simulink model "decoder"  (R2012b)
settings: Solver=FixedStepDiscrete  StartTime=0.0  StopTime=10.0  FixedStep=0.001  RelTol=1e-3
undefined symbols (not defined in the file): A, biasCorrectionEnable, biasCorrectionInitial, biasCorrectionPower, biasCorrectionResetToInitial, biasCorrectionStateInds, biasCorrectionTau, biasCorrectionType, biasCorrectionVelocityThreshold, C, Cfeedback, continuousEnable, DecoderConstants, decoderType, discreteEnable, discreteFilterName, discreteInvSoftNormVals, discretePcaMeans, discreteProjector, dtMS, filterName, gainK, hLFPDivisor, hLFPTransform, hmmEmisCovarDet, hmmEmisCovarInv, hmmEmisMean, hmmNumStates, hmmSpeedScalingBins, hmmSpeedScalingEnable, hmmSpeedScalingPs, hmmStateModel, hmmTrans, invSoftNormVals, K, meansTrackingEnable, meansTrackingInitial, meansTrackingPeriodMS, meansTrackingResetToCurrent, meansTrackingResetToInitial, meansTrackingUseFastAdapt, offsetXk, pcaMeans, projector, scaleXk, smoothingKernel, spikeTransform, thresholds, useAcaus, xkConstants
settings Model: xpc_rtwmakecfg_data=_xpcetherlib__xpcether8255xlib__xpcetherGbElib__xpcnblib_  Creator=gilja  LastModifiedBy=NPTL
settings SolverCC: EnableConcurrentExecution=on  ConcurrentTasks=on
settings DataIOCC: LimitDataPoints=off  SaveOutput=off  SaveTime=off
settings OptimizationCC: InlineParams=on  InlineInvariantSignals=on  EnhancedBackFolding=on  EfficientFloat2IntCast=on  SimCompilerOptimization=On
settings DebuggingCC: IntegerOverflowMsg=none
settings HardwareCC: ProdIntDivRoundTo=Zero  ProdEndianess=LittleEndian  ProdHWDeviceType=Generic->32-bit x86 compatible
settings ModelReferenceCC: ModelReferenceNumInstancesAllowed=Single  ModelReferenceMinAlgLoopOccurrences=on
settings RTWCC: SystemTargetFile=xpctarget.tlc  TemplateMakefile=xpc_default_tmf  Description=xPC Target  ProcessScript=xpctarget_make_rtw_hook  RTWCompilerOptimization=On  RTWCustomCompilerOptimizations=-O fold_scalar_mxarrays:on -O fold_non_scalar_mxarrays:on -O array_indexing:on -O optimize_integer_for_loops:on -O optimize_conditionals:on
settings CodeAppCC: MaxIdLength=62
settings xpcTargetCC: TargetFcnLib=ansi_tfl_table_tmw.mat  CodeReplacementLibrary=XPC_BLAS  ParMdlRefBuildCompliant=on  ConcurrentExecutionCompliant=on  CombineSignalStateStructs=off  GRTInterface=on  ExtMode=off  xPCTaskExecutionProfile=on  xPCRL32EventNumber=5000  xPCisDownloadable=off  xPCLoadParamSetFile=off  xPCConcurrentTasks=off  xPCEnableSFAnimation=off

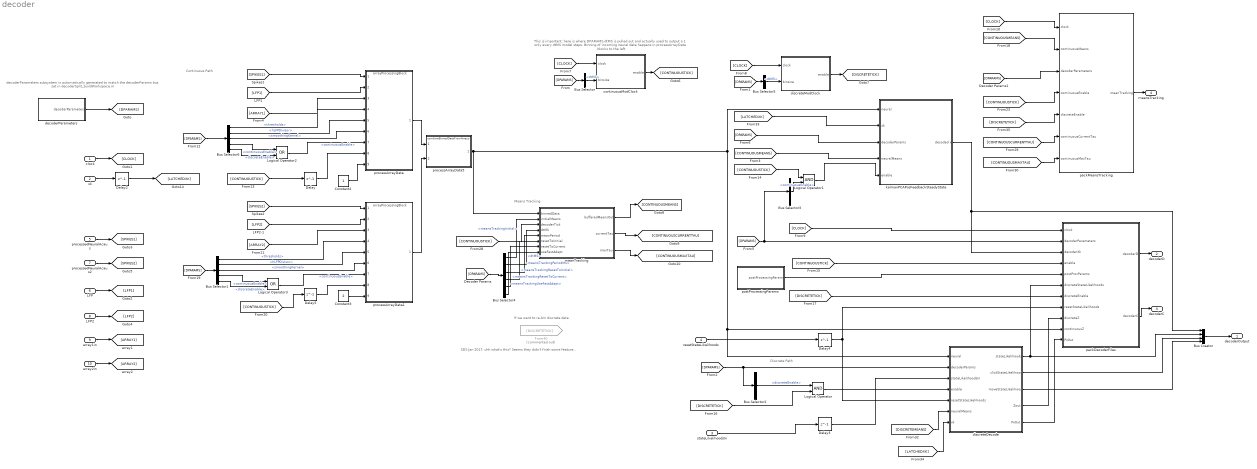
== system decoder ==
  note: SDS Jan 2017: uhh what's this? Seems they didn't fnish some feature...
  note: This is important: here is where DPARAMS.dtMS is pulled out and actually used to
      | output a 1 only every dtMS model steps. Binning of incoming neural data happens in
      | processArrayData blocks to the left
  note: Means Tracking
  note: decoderParameters subsystem is
      |  automatically generated to match the decoderParams
      | bus set in decoderSplit_buildWorkspace.m
  note: Discrete Path
  note: Continuous Path
  note: If we want to re-bin discrete data
  clock : Inport  OutDataTypeStr=uint32
  xk : Inport  Port=2  OutDataTypeStr=double  PortDimensions=[double(xkConstants.NUM_STATE_DIMENSIONS),1]
  stateLikelihoodsIn : Inport  Port=3  OutDataTypeStr=double  PortDimensions=[double(DecoderConstants.MAX_DISCRETE_STATES) 1]
  resetStateLikelihoods : Inport  Port=4  OutDataTypeStr=double  PortDimensions=1
  processedNeuralAcaus : Inport  Port=5  OutDataTypeStr=Bus: processedNeural  BusOutputAsStruct=on
  LFP : Inport  Port=6  OutDataTypeStr=single  PortDimensions=[1 96]
  processedNeuralAcaus2 : Inport  Port=7  OutDataTypeStr=Bus: processedNeural  BusOutputAsStruct=on
  LFP2 : Inport  Port=8  OutDataTypeStr=single  PortDimensions=[1 96]
  array1in : Inport  Port=9  OutDataTypeStr=uint8  BusOutputAsStruct=on
  array2in : Inport  Port=10  OutDataTypeStr=uint8  BusOutputAsStruct=on
  Bus Creator : BusCreator  OutDataTypeStr=Bus: decoderOutput  NonVirtualBus=on
  Bus Selector : BusSelector  OutputSignals=dtMS
  Bus Selector1 : BusSelector  OutputSignals=thresholds,hLFPDivisor,smoothingKernel,continuousEnable,discreteEnable
  Bus Selector2 : BusSelector  OutputSignals=discreteEnable
  Bus Selector3 : BusSelector  OutputSignals=continuousEnable
  Bus Selector4 : BusSelector  OutputSignals=meansTrackingInitial,dtMS,meansTrackingPeriodMS,meansTrackingResetToInitial,meansTrackingResetToCurrent,meansTrackingUseFastAdapt
  Bus Selector5 : BusSelector  OutputSignals=dtMS
  Bus Selector6 : BusSelector  OutputSignals=thresholds,hLFPDivisor,smoothingKernel,continuousEnable,discreteEnable
  Constant2 : Constant  VectorParams1D=off  SampleTime=-1
  Constant3 : Constant  Value=2  VectorParams1D=off  SampleTime=-1
  Delay{,2..5} (5 alike) : Delay  DelayLength=1
  From40 : From  Commented=on  GotoTag=DISCRETETICK
  Logical Operator : Logic  AllPortsSameDT=off  OutDataTypeStr=boolean
  Logical Operator1 : Logic  AllPortsSameDT=off  OutDataTypeStr=boolean
  Logical Operator2 : Logic  Operator=OR  AllPortsSameDT=off  OutDataTypeStr=boolean
  Logical Operator3 : Logic  Operator=OR  AllPortsSameDT=off  OutDataTypeStr=boolean
  continuousModClock : MATLAB Function  TreatAsAtomicUnit=on
  decoderParameters : Subsystem
  discreteDecode : Subsystem
  discreteModClock : MATLAB Function  TreatAsAtomicUnit=on
  kalmanPCAPosFeedbackSteadyState : Subsystem
  meanTracking : MATLAB Function  TreatAsAtomicUnit=on
  packDecoderFiles : MATLAB Function  TreatAsAtomicUnit=on
  packMeansTracking : MATLAB Function  TreatAsAtomicUnit=on
  postProcessingParams : Subsystem
  processArrayData : ModelReference  ModelNameDialog=arrayProcessingBlock  SimulationMode=Normal  ModelReferenceVersion=1.56  CopyOfModelName=arrayProcessingBlock  DefaultDataLogging=on
  processArrayData1 : ModelReference  ModelNameDialog=arrayProcessingBlock  SimulationMode=Normal  ModelReferenceVersion=1.56  CopyOfModelName=arrayProcessingBlock  DefaultDataLogging=on
  processArrayData5 : ModelReference  ModelNameDialog=combineBinnedDataFromArrays  SimulationMode=Normal  ModelReferenceVersion=1.49  CopyOfModelName=combineBinnedDataFromArrays  DefaultDataLogging=on
  decoderOutput : Outport  OutDataTypeStr=Bus: decoderOutput  BusOutputAsStruct=on
  decoderD : Outport  Port=2  OutDataTypeStr=Bus: fileLoggerFormatAndData  BusOutputAsStruct=on
  decoderC : Outport  Port=3  OutDataTypeStr=Bus: fileLoggerFormatAndData  BusOutputAsStruct=on
  meansTracking : Outport  Port=4  OutDataTypeStr=Bus: fileLoggerFormatAndData  BusOutputAsStruct=on
  wires:
  Bus Selector/1 -> continuousModClock/2(binsize)  "<dtMS>"
  [LATCHEDXK] -> kalmanPCAPosFeedbackSteadyState/2(xk)
  decoderParameters/1(decoderParameters) -> [DPARAMS]
  discreteDecode/1(stateLikelihoods) -> Bus Creator/2, packDecoderFiles/6(discreteStateLikelihoods)
  Bus Creator/1 -> decoderOutput/1
  stateLikelihoodsIn/1 -> Delay3/1
  Delay3/1 -> discreteDecode/3(stateLikelihoodsIn)
  discreteDecode/2(clickStateLikelihood) -> Bus Creator/3
  discreteDecode/3(moveStateLikelihood) -> Bus Creator/4
  Delay4/1 -> discreteDecode/5(resetStateLikelihoods), packDecoderFiles/8(resetStateLikelihoods)
  resetStateLikelihoods/1 -> Delay4/1
  [DPARAMS] -> Bus Selector/1
  [DPARAMS] -> Bus Selector2/1, discreteDecode/2(decoderParams)
  [DPARAMS] -> kalmanPCAPosFeedbackSteadyState/3(decoderParams)
  clock/1 -> [CLOCK]
  [CLOCK] -> continuousModClock/1(clock)
  [CLOCK] -> packDecoderFiles/1(clock)
  LFP/1 -> [LFP1]
  processedNeuralAcaus/1 -> [SPIKES1]
  discreteDecode/4(Zout) -> packDecoderFiles/9(discreteZ)
  LFP2/1 -> [LFP2]
  processedNeuralAcaus2/1 -> [SPIKES2]
  array1in/1 -> [ARRAY1]
  array2in/1 -> [ARRAY2]
  [DPARAMS] -> Bus Selector6/1
  [SPIKES1] -> processArrayData/1
  [LFP1] -> processArrayData/2
  Bus Selector6/2 -> processArrayData/5  "<hLFPDivisor>"
  Bus Selector6/3 -> processArrayData/6  "<smoothingKernel>"
  Delay/1 -> processArrayData/8
  [ARRAY1] -> processArrayData/3
  continuousModClock/1(enable) -> [CONTINUOUSTICK]
  [CONTINUOUSTICK] -> Delay/1
  [CONTINUOUSTICK] -> packDecoderFiles/4(enable)
  Logical Operator/1 -> discreteDecode/4(enable)
  [DISCRETETICK] -> packDecoderFiles/7(discreteEnable)
  [DPARAMS] -> Bus Selector1/1
  [SPIKES2] -> processArrayData1/1
  [LFP2] -> processArrayData1/2
  Bus Selector1/2 -> processArrayData1/5  "<hLFPDivisor>"
  Bus Selector1/3 -> processArrayData1/6  "<smoothingKernel>"
  Delay5/1 -> processArrayData1/8
  [ARRAY2] -> processArrayData1/3
  [CONTINUOUSTICK] -> Delay5/1
  processArrayData/1 -> processArrayData5/1
  processArrayData1/1 -> processArrayData5/2
  Constant2/1 -> processArrayData/9
  Bus Selector6/1 -> processArrayData/4  "<thresholds>"
  Bus Selector1/1 -> processArrayData1/4  "<thresholds>"
  Constant3/1 -> processArrayData1/9
  [CLOCK] -> discreteModClock/1(clock)
  discreteModClock/1(enable) -> [DISCRETETICK]
  Logical Operator3/1 -> processArrayData1/7  "<continuousEnable>"
  Logical Operator2/1 -> processArrayData/7  "<continuousEnable>"
  [DISCRETETICK] -> Logical Operator/2
  Bus Selector2/1 -> Logical Operator/1  "<discreteEnable>"
  Bus Selector3/1 -> Logical Operator1/2  "<continuousEnable>"
  Logical Operator1/1 -> kalmanPCAPosFeedbackSteadyState/5(enable)
  [CONTINUOUSTICK] -> Logical Operator1/1
  [DPARAMS] -> Bus Selector3/1, packDecoderFiles/2(decoderParameters)
  [DPARAMS] -> Bus Selector4/1
  Bus Selector4/2 -> meanTracking/4(dtMS)  "<dtMS>"
  Bus Selector4/1 -> meanTracking/2(initialMeans)  "<meansTrackingInitial>"
  meanTracking/1(bufferedMeansOut) -> [CONTINUOUSMEANS]
  [CONTINUOUSMEANS] -> kalmanPCAPosFeedbackSteadyState/4(neuralMeans)
  [CLOCK] -> packMeansTracking/1(clock)
  [DPARAMS] -> packMeansTracking/3(decoderParameters)
  [CONTINUOUSMEANS] -> packMeansTracking/2(continuousMeans)
  [CONTINUOUSTICK] -> packMeansTracking/4(continuousEnable)
  [CONTINUOUSTICK] -> meanTracking/3(decoderTick)
  Bus Selector4/3 -> meanTracking/5(meanPeriod)  "<meansTrackingPeriodMS>"
  Bus Selector4/4 -> meanTracking/6(resetToInitial)  "<meansTrackingResetToInitial>"
  Bus Selector4/5 -> meanTracking/7(resetToCurrent)  "<meansTrackingResetToCurrent>"
  Bus Selector4/6 -> meanTracking/8(useFastAdapt)  "<meansTrackingUseFastAdapt>"
  meanTracking/2(currentTau) -> [CONTINUOUSCURRENTTAU]
  meanTracking/3(maxTau) -> [CONTINUOUSMAXTAU]
  [CONTINUOUSMAXTAU] -> packMeansTracking/7(continuousMaxTau)
  [CONTINUOUSCURRENTTAU] -> packMeansTracking/6(continuousCurrentTau)
  processArrayData5/1 -> meanTracking/1(binnedData), discreteDecode/1(neural), packDecoderFiles/10(continuousZ), kalmanPCAPosFeedbackSteadyState/1(neural)
  [DISCRETEMEANS] -> discreteDecode/6(neuralMeans)
  [LATCHEDXK] -> discreteDecode/7(xk)
  Delay2/1 -> [LATCHEDXK]
  xk/1 -> Delay2/1
  [DISCRETETICK] -> packMeansTracking/5(discreteEnable)
  kalmanPCAPosFeedbackSteadyState/1(decoded x) -> packDecoderFiles/3(decoderXk), Bus Creator/1
  Bus Selector6/4 -> Logical Operator2/1  "<continuousEnable>"
  Bus Selector6/5 -> Logical Operator2/2  "<discreteEnable>"
  Bus Selector1/4 -> Logical Operator3/1  "<continuousEnable>"
  Bus Selector1/5 -> Logical Operator3/2  "<discreteEnable>"
  packMeansTracking/1(meanTracking) -> meansTracking/1
  packDecoderFiles/2(decoderC) -> decoderC/1
  packDecoderFiles/1(decoderD) -> decoderD/1
  Bus Selector5/1 -> discreteModClock/2(binsize)  "<dtMS>"
  [DPARAMS] -> Bus Selector5/1
  discreteDecode/5(PxOut) -> packDecoderFiles/11(PxOut)
  postProcessingParams/1(postProcessingParams) -> packDecoderFiles/5(postProcParams)

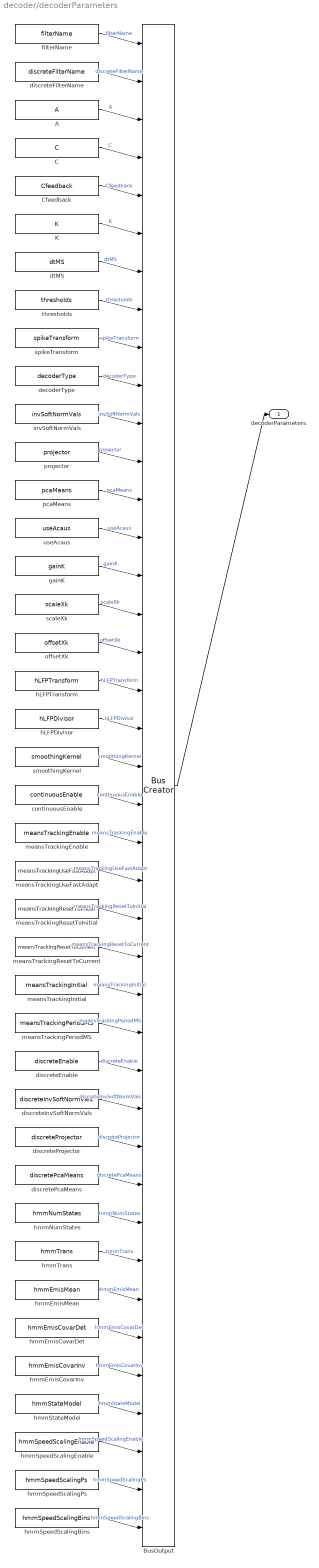
== system decoder/decoderParameters ==
  A : Constant  Value=A
  BusOutput : BusCreator  Inputs=filterName,discreteFilterName,A,C,Cfeedback,K,dtMS,thresholds,spikeTransform,decoderType,invSoftNormVals,projector,pcaMeans,useAcaus,gainK,scaleXk,offsetXk,hLFPTransform,hLFPDivisor,smoothingKernel,continuousEnable,meansTrackingEnable,meansTrackingUseFastAdapt,meansTrackingResetToInitial,meansTrackingResetToCurrent,meansTrackingInitial,meansTrackingPeriodMS,discreteEnable,discreteInvSoftNormVals,discreteProjector,discretePcaMeans,hmmNumStates,hmmTrans,hmmEmisMean,hmmEmisCovarDet,hmmEmisCovarInv,hmmStateModel,hmmSpeedScalingEnable,hmmSpeedScalingPs,hmmSpeedScalingBins  OutDataTypeStr=Bus: decoderParams
  C : Constant  Value=C
  Cfeedback : Constant  Value=Cfeedback
  K : Constant  Value=K
  continuousEnable : Constant  Value=continuousEnable
  decoderType : Constant  Value=decoderType
  discreteEnable : Constant  Value=discreteEnable
  discreteFilterName : Constant  Value=discreteFilterName
  discreteInvSoftNormVals : Constant  Value=discreteInvSoftNormVals
  discretePcaMeans : Constant  Value=discretePcaMeans
  discreteProjector : Constant  Value=discreteProjector
  dtMS : Constant  Value=dtMS
  filterName : Constant  Value=filterName
  gainK : Constant  Value=gainK
  hLFPDivisor : Constant  Value=hLFPDivisor
  hLFPTransform : Constant  Value=hLFPTransform
  hmmEmisCovarDet : Constant  Value=hmmEmisCovarDet
  hmmEmisCovarInv : Constant  Value=hmmEmisCovarInv
  hmmEmisMean : Constant  Value=hmmEmisMean
  hmmNumStates : Constant  Value=hmmNumStates
  hmmSpeedScalingBins : Constant  Value=hmmSpeedScalingBins
  hmmSpeedScalingEnable : Constant  Value=hmmSpeedScalingEnable
  hmmSpeedScalingPs : Constant  Value=hmmSpeedScalingPs
  hmmStateModel : Constant  Value=hmmStateModel
  hmmTrans : Constant  Value=hmmTrans
  invSoftNormVals : Constant  Value=invSoftNormVals
  meansTrackingEnable : Constant  Value=meansTrackingEnable
  meansTrackingInitial : Constant  Value=meansTrackingInitial
  meansTrackingPeriodMS : Constant  Value=meansTrackingPeriodMS
  meansTrackingResetToCurrent : Constant  Value=meansTrackingResetToCurrent
  meansTrackingResetToInitial : Constant  Value=meansTrackingResetToInitial
  meansTrackingUseFastAdapt : Constant  Value=meansTrackingUseFastAdapt
  offsetXk : Constant  Value=offsetXk
  pcaMeans : Constant  Value=pcaMeans
  projector : Constant  Value=projector
  scaleXk : Constant  Value=scaleXk
  smoothingKernel : Constant  Value=smoothingKernel
  spikeTransform : Constant  Value=spikeTransform
  thresholds : Constant  Value=thresholds
  useAcaus : Constant  Value=useAcaus
  decoderParameters : Outport
  wires:
  filterName/1 -> BusOutput/1  "filterName"
  discreteFilterName/1 -> BusOutput/2  "discreteFilterName"
  A/1 -> BusOutput/3  "A"
  C/1 -> BusOutput/4  "C"
  Cfeedback/1 -> BusOutput/5  "Cfeedback"
  K/1 -> BusOutput/6  "K"
  dtMS/1 -> BusOutput/7  "dtMS"
  thresholds/1 -> BusOutput/8  "thresholds"
  spikeTransform/1 -> BusOutput/9  "spikeTransform"
  decoderType/1 -> BusOutput/10  "decoderType"
  invSoftNormVals/1 -> BusOutput/11  "invSoftNormVals"
  projector/1 -> BusOutput/12  "projector"
  pcaMeans/1 -> BusOutput/13  "pcaMeans"
  useAcaus/1 -> BusOutput/14  "useAcaus"
  gainK/1 -> BusOutput/15  "gainK"
  scaleXk/1 -> BusOutput/16  "scaleXk"
  offsetXk/1 -> BusOutput/17  "offsetXk"
  hLFPTransform/1 -> BusOutput/18  "hLFPTransform"
  hLFPDivisor/1 -> BusOutput/19  "hLFPDivisor"
  smoothingKernel/1 -> BusOutput/20  "smoothingKernel"
  continuousEnable/1 -> BusOutput/21  "continuousEnable"
  meansTrackingEnable/1 -> BusOutput/22  "meansTrackingEnable"
  meansTrackingUseFastAdapt/1 -> BusOutput/23  "meansTrackingUseFastAdapt"
  meansTrackingResetToInitial/1 -> BusOutput/24  "meansTrackingResetToInitial"
  meansTrackingResetToCurrent/1 -> BusOutput/25  "meansTrackingResetToCurrent"
  meansTrackingInitial/1 -> BusOutput/26  "meansTrackingInitial"
  meansTrackingPeriodMS/1 -> BusOutput/27  "meansTrackingPeriodMS"
  discreteEnable/1 -> BusOutput/28  "discreteEnable"
  discreteInvSoftNormVals/1 -> BusOutput/29  "discreteInvSoftNormVals"
  discreteProjector/1 -> BusOutput/30  "discreteProjector"
  discretePcaMeans/1 -> BusOutput/31  "discretePcaMeans"
  hmmNumStates/1 -> BusOutput/32  "hmmNumStates"
  hmmTrans/1 -> BusOutput/33  "hmmTrans"
  hmmEmisMean/1 -> BusOutput/34  "hmmEmisMean"
  hmmEmisCovarDet/1 -> BusOutput/35  "hmmEmisCovarDet"
  hmmEmisCovarInv/1 -> BusOutput/36  "hmmEmisCovarInv"
  hmmStateModel/1 -> BusOutput/37  "hmmStateModel"
  hmmSpeedScalingEnable/1 -> BusOutput/38  "hmmSpeedScalingEnable"
  hmmSpeedScalingPs/1 -> BusOutput/39  "hmmSpeedScalingPs"
  hmmSpeedScalingBins/1 -> BusOutput/40  "hmmSpeedScalingBins"
  BusOutput/1 -> decoderParameters/1

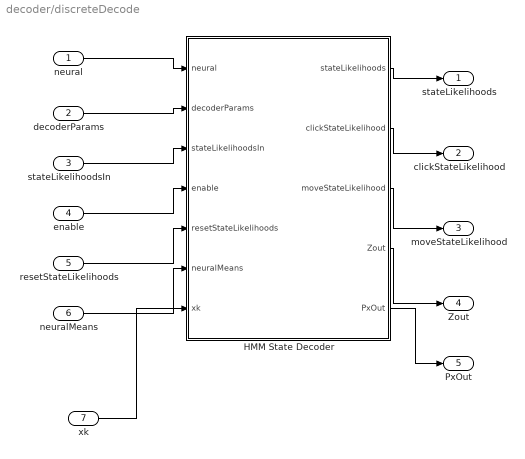
== system decoder/discreteDecode ==
  neural : Inport
  decoderParams : Inport  Port=2
  stateLikelihoodsIn : Inport  Port=3
  enable : Inport  Port=4
  resetStateLikelihoods : Inport  Port=5
  neuralMeans : Inport  Port=6
  xk : Inport  Port=7
  HMM State Decoder : Subsystem
  stateLikelihoods : Outport
  clickStateLikelihood : Outport  Port=2
  moveStateLikelihood : Outport  Port=3
  Zout : Outport  Port=4
  PxOut : Outport  Port=5
  wires:
  enable/1 -> HMM State Decoder/4(enable)
  decoderParams/1 -> HMM State Decoder/2(decoderParams)
  neural/1 -> HMM State Decoder/1(neural)
  HMM State Decoder/2(clickStateLikelihood) -> clickStateLikelihood/1
  HMM State Decoder/3(moveStateLikelihood) -> moveStateLikelihood/1
  HMM State Decoder/1(stateLikelihoods) -> stateLikelihoods/1
  stateLikelihoodsIn/1 -> HMM State Decoder/3(stateLikelihoodsIn)
  resetStateLikelihoods/1 -> HMM State Decoder/5(resetStateLikelihoods)
  HMM State Decoder/4(Zout) -> Zout/1
  neuralMeans/1 -> HMM State Decoder/6(neuralMeans)
  xk/1 -> HMM State Decoder/7(xk)
  HMM State Decoder/5(PxOut) -> PxOut/1

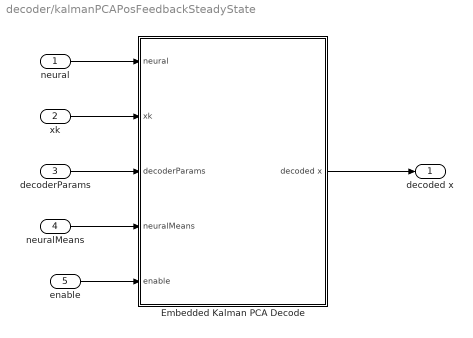
== system decoder/kalmanPCAPosFeedbackSteadyState ==
  neural : Inport
  xk : Inport  Port=2
  decoderParams : Inport  Port=3
  neuralMeans : Inport  Port=4
  enable : Inport  Port=5
  Embedded Kalman PCA Decode : Subsystem
  decoded x : Outport
  wires:
  enable/1 -> Embedded Kalman PCA Decode/5(enable)
  decoderParams/1 -> Embedded Kalman PCA Decode/3(decoderParams)
  xk/1 -> Embedded Kalman PCA Decode/2(xk)
  neural/1 -> Embedded Kalman PCA Decode/1(neural)
  Embedded Kalman PCA Decode/1(decoded x) -> decoded x/1
  neuralMeans/1 -> Embedded Kalman PCA Decode/4(neuralMeans)

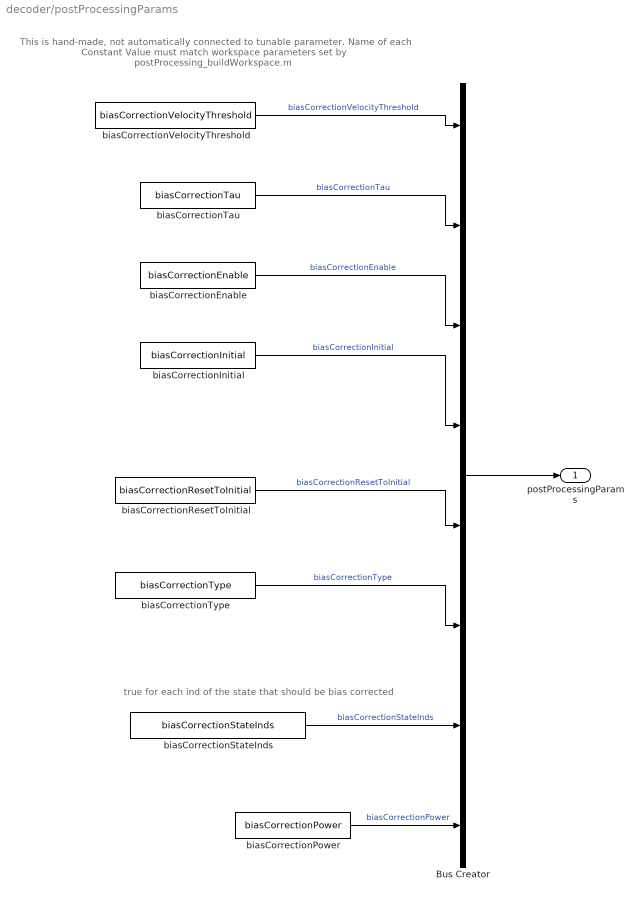
== system decoder/postProcessingParams ==
  note: true for each ind of the state that should be bias corrected
  note: This is hand-made, not automatically connected to tunable parameter.
      | Name of each Constant Value must match workspace parameters set by
      | postProcessing_buildWorkspace.m
  Bus Creator : BusCreator  Inputs=8  OutDataTypeStr=Bus: postProcessingParams  NonVirtualBus=on
  biasCorrectionEnable : Constant  Value=biasCorrectionEnable
  biasCorrectionInitial : Constant  Value=biasCorrectionInitial
  biasCorrectionPower : Constant  Value=biasCorrectionPower
  biasCorrectionResetToInitial : Constant  Value=biasCorrectionResetToInitial
  biasCorrectionStateInds : Constant  Value=biasCorrectionStateInds
  biasCorrectionTau : Constant  Value=biasCorrectionTau
  biasCorrectionType : Constant  Value=biasCorrectionType
  biasCorrectionVelocityThreshold : Constant  Value=biasCorrectionVelocityThreshold
  postProcessingParams : Outport
  wires:
  Bus Creator/1 -> postProcessingParams/1
  biasCorrectionVelocityThreshold/1 -> Bus Creator/1  "biasCorrectionVelocityThreshold"
  biasCorrectionEnable/1 -> Bus Creator/3  "biasCorrectionEnable"
  biasCorrectionTau/1 -> Bus Creator/2  "biasCorrectionTau"
  biasCorrectionInitial/1 -> Bus Creator/4  "biasCorrectionInitial"
  biasCorrectionResetToInitial/1 -> Bus Creator/5  "biasCorrectionResetToInitial"
  biasCorrectionType/1 -> Bus Creator/6  "biasCorrectionType"
  biasCorrectionStateInds/1 -> Bus Creator/7  "biasCorrectionStateInds"
  biasCorrectionPower/1 -> Bus Creator/8  "biasCorrectionPower"

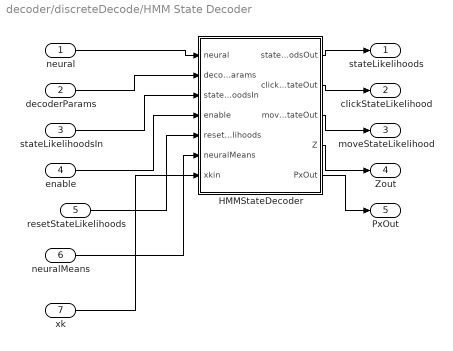
== system decoder/discreteDecode/HMM State Decoder ==
  neural : Inport
  decoderParams : Inport  Port=2
  stateLikelihoodsIn : Inport  Port=3
  enable : Inport  Port=4
  resetStateLikelihoods : Inport  Port=5
  neuralMeans : Inport  Port=6
  xk : Inport  Port=7
  HMMStateDecoder : MATLAB Function  TreatAsAtomicUnit=on
  stateLikelihoods : Outport
  clickStateLikelihood : Outport  Port=2
  moveStateLikelihood : Outport  Port=3
  Zout : Outport  Port=4
  PxOut : Outport  Port=5
  wires:
  enable/1 -> HMMStateDecoder/4(enable)
  decoderParams/1 -> HMMStateDecoder/2(decoderParams)
  neural/1 -> HMMStateDecoder/1(neural)
  HMMStateDecoder/2(clickStateOut) -> clickStateLikelihood/1
  HMMStateDecoder/3(moveStateOut) -> moveStateLikelihood/1
  HMMStateDecoder/1(stateLikelihoodsOut) -> stateLikelihoods/1
  stateLikelihoodsIn/1 -> HMMStateDecoder/3(stateLikelihoodsIn)
  resetStateLikelihoods/1 -> HMMStateDecoder/5(resetStateLikelihoods)
  HMMStateDecoder/4(Z) -> Zout/1
  neuralMeans/1 -> HMMStateDecoder/6(neuralMeans)
  xk/1 -> HMMStateDecoder/7(xkin)
  HMMStateDecoder/5(PxOut) -> PxOut/1

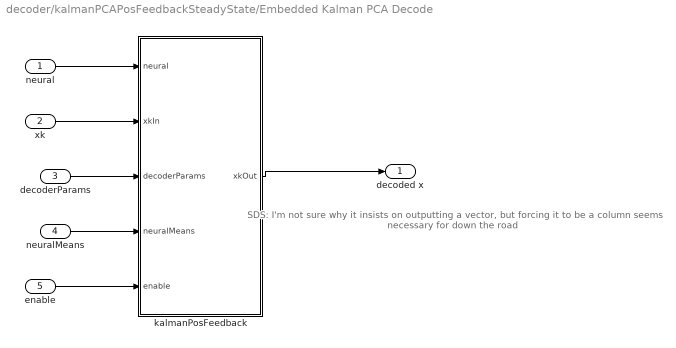
== system decoder/kalmanPCAPosFeedbackSteadyState/Embedded Kalman PCA Decode ==
  note: SDS: I'm not sure why it insists on outputting a vector, but forcing it to
      | be a column seems necessary for down the road
  neural : Inport
  xk : Inport  Port=2
  decoderParams : Inport  Port=3
  neuralMeans : Inport  Port=4
  enable : Inport  Port=5
  kalmanPosFeedback : MATLAB Function  TreatAsAtomicUnit=on
  decoded x : Outport
  wires:
  enable/1 -> kalmanPosFeedback/5(enable)
  decoderParams/1 -> kalmanPosFeedback/3(decoderParams)
  neural/1 -> kalmanPosFeedback/1(neural)
  xk/1 -> kalmanPosFeedback/2(xkIn)
  neuralMeans/1 -> kalmanPosFeedback/4(neuralMeans)
  kalmanPosFeedback/1(xkOut) -> decoded x/1

== matlab function decoder/meanTracking ==
  data: binnedData input; bufferedMeansOut output; initialMeans input; decoderTick input; dtMS input; meanPeriod input; resetToInitial input; resetToCurrent input; useFastAdapt input; currentTau output; maxTau output
function [bufferedMeansOut,currentTau,maxTau] = meanTracking(binnedData, initialMeans, decoderTick, dtMS, meanPeriod, resetToInitial, resetToCurrent, useFastAdapt)
%#codegen
persistent bufferedMeans currentT;

% currentT is the time since last reset

if isempty(bufferedMeans) || resetToCurrent
    bufferedMeans = double(binnedData(:) / double(dtMS));
    currentT = uint16(0);
end

maxTau = double(meanPeriod);
useTau = maxTau;

if resetToInitial
    bufferedMeans = double(initialMeans(:));
    currentT = uint16(0);
end

if decoderTick
    currentT = uint16(currentT) + uint16(dtMS);

    % if fast-adapting - tau adjusts, to give most recent data priority.
    % adjustment maxes out at the desired "meanPeriod"
    if useFastAdapt
        useTau = min(useTau, double(currentT));
    end
    
    % here is the actual mean tracking
    % each decoder tick has the weight of one bin width (i.e. a 50ms bin
    % should count for 50 values)
    %% if tau == 0 , disable mean tracking
    if useTau
        bufferedMeans = bufferedMeans(:) + (double(binnedData(:))  - bufferedMeans(:)*double(dtMS)) / useTau;
    end
end

bufferedMeansOut = bufferedMeans(:);
currentTau = useTau;
end

== matlab function decoder/packMeansTracking ==
  data: clock input uint32; continuousMeans input double; decoderParameters input Bus: decoderParams; meanTracking output Bus: fileLoggerFormatAndData; continuousEnable input; discreteEnable input; continuousCurrentTau input; continuousMaxTau input
function meanTracking  = packMeansTracking(clock, continuousMeans, decoderParameters, continuousEnable, discreteEnable, continuousCurrentTau, continuousMaxTau)

%CP/PN - removing discrete means tracking
%function meanTracking  = packMeansTracking(clock, continuousMeans, discreteMeans, decoderParameters, continuousEnable, discreteEnable, continuousCurrentTau, continuousMaxTau)

%#codegen
    
VERSION_ID = zeros([1 1],'uint16');
VERSION_ID(1) = uint16(2);

persistent iContCurr;
%persistent iDiscCurr;

if isempty(iContCurr)
    iContCurr = uint16(1);
%    iDiscCurr = uint16(1);
else
    iContCurr = iContCurr+uint16(2);
%    iDiscCurr = iDiscCurr+uint16(2);
end

if iContCurr+1 > numel(continuousMeans)
    iContCurr = uint16(1);
end
%if iDiscCurr+1 > numel(discreteMeans)
%    iDiscCurr = uint16(1);
%end


%% PACK DATA FOR UDP OUTPUT
meanTracking = packFileLoggerFormatAndData('meanTracking', ...
    'version', VERSION_ID, ...
    'clock', clock, ...
    'contMean1Ind', iContCurr, ...
    'contMean2Ind', iContCurr+1, ...
    'contMean1Val', single(continuousMeans(iContCurr)), ...
    'contMean2Val', single(continuousMeans(iContCurr+1)), ...
    'continuousResetToInitial', logical(decoderParameters.meansTrackingResetToInitial), ...
    'continuousResetToCurrent', logical(decoderParameters.meansTrackingResetToCurrent), ...
    'continuousEnable', logical(decoderParameters.meansTrackingEnable), ...
    'continuousCurrentTau', single(continuousCurrentTau), ...
    'continuousMaxTau', single(continuousMaxTau) ...
);


%     'discMean1Ind', iDiscCurr, ...
%     'discMean2Ind', iDiscCurr+1, ...
%     'discMean1Val', single(discreteMeans(iDiscCurr)), ...
%     'discMean2Val', single(discreteMeans(iDiscCurr+1)), ...

meanTracking.data.send = logical(continuousEnable); % send means tracking only if enabled

== matlab function decoder/continuousModClock ==
  data: clock input; binsize input; enable output
function enable = moduloClock(clock, binsize)
    persistent enableOut
    if isempty(enableOut)
        enableOut = 0;
    end
    
    modded = mod(double(clock), double(binsize));
    
    if any(modded(:))
        enableOut = 0;
    else
        enableOut = 1;
    end
    
    enable = enableOut;

== matlab function decoder/kalmanPCAPosFeedbackSteadyState/Embedded Kalman PCA Decode/kalmanPosFeedback ==
  data: neural input size=[1 uint16(DecoderConstants.NUM_CONTINUOUS_CHANNELS)]; xkIn input; xkOut output size=[double(xkConstants.NUM_STATE_DIMENSIONS),1]; decoderParams input Bus: decoderParams; neuralMeans input; enable input
function xkOut = kalmanPosFeedback(neural, xkIn, decoderParams, neuralMeans, enable )
%codgen
%% steady state kalman filter

% xkInFull is the Nx1 (e.g. 20x1).
STATEVEC_SIZE = double(xkConstants.NUM_STATE_DIMENSIONS); 

persistent xk;
xkIn(end) = 1; % we always want and assume that the last element of xk is 1s, so we
               % can use it as a bias. This should be set by updateXk too,
               % but just in case that gets changed in some future code
               % update, do it here too.
if(isempty(xk))
    xk = xkIn;
end

A = decoderParams.A; % this is actually A, NOT M1
C = decoderParams.C; % This is C
K = decoderParams.K; % this is K from steady state. That's the key reason thsi code works and is truly a 
                     % steady-state Kalman. AKA "M2" in rigC parlance.
Cfeedback = decoderParams.Cfeedback; % This is Cfeedback.
dtMS = decoderParams.dtMS;

spikeTransform = decoderParams.spikeTransform;
decoderType = decoderParams.decoderType;
invSoftNormVals = decoderParams.invSoftNormVals;
meansTrackingEnable = decoderParams.meansTrackingEnable;

gainK = decoderParams.gainK;
scaleXk = decoderParams.scaleXk;
offsetXk = decoderParams.offsetXk;

pcaMeans = decoderParams.pcaMeans;
projector = decoderParams.projector;


if enable
    
    % Position has already been updated by the task, just need the prior on
    % velocity to be updated
    xk = xkIn./scaleXk; %undo scaling so internal xK is sized "true"
    xk(2:2:STATEVEC_SIZE) = A(2:2:STATEVEC_SIZE, 2:2:STATEVEC_SIZE)*xk(2:2:STATEVEC_SIZE);
    
    %% transform "neural" data for some decoders
    switch decoderType
        case DecoderConstants.DECODER_TYPE_VFBSSKF
            %xk = xk + gainK.*(K*(neural(:)-C*xk));
        case DecoderConstants.DECODER_TYPE_VFBNORMSSKF
            neural(:) = neural(:) .* invSoftNormVals;
            neuralMeans(:) = neuralMeans(:) .* invSoftNormVals;
        case DecoderConstants.DECODER_TYPE_PCAVFBSSKF
            neural(:) = neural(:) .* invSoftNormVals;
            neuralMeans(:) = neuralMeans(:) .* invSoftNormVals;
    end

    if meansTrackingEnable
        % effectively zeroing out the bias term in C
        % This is important, otherwise with meansTracking we'd be
        % subtracting two different biases from the neural data (one from
        % neuralMeans, the other from the offset term of C), and thus most
        % likely introducting another bias
        xk(STATEVEC_SIZE) = 0;
        neural(:) = neural(:) - neuralMeans(:) * double(dtMS);
    else
        if decoderType == DecoderConstants.DECODER_TYPE_PCAVFBSSKF
            neural(:) = neural(:) - pcaMeans;
        end
    end
    
    % apply Cfeedback operation to neural.
    neural(:) = neural(:) - Cfeedback*xk.*invSoftNormVals;
    
    % up to this point, "neural" should be a single
    
    switch decoderType
        case {DecoderConstants.DECODER_TYPE_VFBSSKF, DecoderConstants.DECODER_TYPE_VFBNORMSSKF}
            xk = xk + gainK.*(K*(double(neural(:))-C*xk));
        case DecoderConstants.DECODER_TYPE_PCAVFBSSKF
            projN = double(projector') * double(neural(:));
            xk = xk + gainK.*(K*(projN-C*xk));
    end
    xk = xk + offsetXk;
    
    xk = scaleXk.*xk; %scale it 
    
end
% output needs to be full-size, with decoded elements expanded into it from
% xk.
xk(end) = 1; % keep 1s here, even if we temporarily disabled due to meansTrackingEnable
xkOut = xk; 

end

== matlab function decoder/packDecoderFiles ==
  data: clock input uint32; decoderParameters input Bus: decoderParams; decoderXk input double; enable input double size=1; decoderD output Bus: fileLoggerFormatAndData; decoderC output Bus: fileLoggerFormatAndData; postProcParams input Bus: postProcessingParams; discreteStateLikelihoods input; discreteEnable input; resetStateLikelihoods input; discreteZ input; continuousZ input; PxOut input
function [decoderD, decoderC] = packNeural(clock, decoderParameters, decoderXk, enable, postProcParams, discreteStateLikelihoods, discreteEnable, resetStateLikelihoods, discreteZ, continuousZ, PxOut)
%#codegen
persistent lastDecoderParameters 

if(isempty(lastDecoderParameters))
    lastDecoderParameters = decoderParameters;
    lastDecoderParameters.filterName = uint8(zeros(1,100)); % force first write
    lastDecoderParameters.discreteFilterName = uint8(zeros(1,100)); % force first write
    lastPPParams = postProcParams;
end

VERSION_ID = zeros([1 1],'uint16');
VERSION_ID(1) = uint16(2);

%% PACK DATA FOR UDP OUTPUT
decoderD = packFileLoggerFormatAndData('decoderD', ...
    'decoderD', VERSION_ID, ...
    'clock', clock, ...
    'filterName', char(decoderParameters.filterName(1:100)), ...
    'discreteFilterName', char(decoderParameters.discreteFilterName(1:100)), ...
    'gainK', decoderParameters.gainK, ...
    'scaleXk', decoderParameters.scaleXk, ...
    'offsetXk', decoderParameters.offsetXk, ...
    'biasCorrVThresh', postProcParams.biasCorrectionVelocityThreshold, ...
    'biasCorrTau', postProcParams.biasCorrectionTau, ...
    'biasCorrType', postProcParams.biasCorrectionType, ...
    'biasCorrEnable', postProcParams.biasCorrectionEnable ...
);

%% this comparison somehow eats 100us ever 100ms. Go fucking figure.
% if((all(lastDecoderParameters.filterName == decoderParameters.filterName)) ...
%         && (all(lastDecoderParameters.discreteFilterName == decoderParameters.discreteFilterName)) ...
%         && (all(lastDecoderParameters.gainK == decoderParameters.gainK)) ...
%         && (all(lastDecoderParameters.offsetXk == decoderParameters.offsetXk)) ...
%         && (all(lastDecoderParameters.scaleXk == decoderParameters.scaleXk)) ...
%         && (all(lastPPParams.biasCorrectionVelocityThreshold == postProcParams.biasCorrectionVelocityThreshold)) ...
%         && (all(lastPPParams.biasCorrectionTau == postProcParams.biasCorrectionTau)) ...
%         && (all(lastPPParams.biasCorrectionEnable == postProcParams.biasCorrectionEnable)))
%     decoderD.data.send = false;
% else
% end

PACKET_OUTPUT_PERIOD = 10000;
if mod(clock, PACKET_OUTPUT_PERIOD)==0
    decoderD.data.send = true;
else
    decoderD.data.send = false;
end    

lastDecoderParameters = decoderParameters;
lastPPParams = postProcParams;

% for now only write out 3 discrete states, obv increase if we have more states
% SNF: we now have more states, write *all* states. There are only like 6 max atm
%ds = zeros([2 1],'single');
ds = zeros([6 1],'single');
ds = single(discreteStateLikelihoods);

decoderC = packFileLoggerFormatAndData('decoderC', ...
    'decoderC', VERSION_ID, ...
    'clock', clock, ...
    'decoderXk', single(decoderXk), ...
    'discreteStateLikelihoods', single(ds), ...
    'resetStateLikelihoods', uint8(resetStateLikelihoods),...
    'decoderEnable', enable, ...
    'discreteZ', discreteZ, ...
    'PxOut', PxOut, ...
    'continuousZ', continuousZ(1:20), ...
    'decoderDiscreteEnable', discreteEnable ...
    );

decoderC.data.send = true;

== matlab function decoder/discreteModClock ==
  data: clock input; binsize input; enable output
function enable = moduloClock(clock, binsize)
    persistent enableOut
    if isempty(enableOut)
        enableOut = 0;
    end
    
    modded = mod(double(clock), double(binsize));
    
    if any(modded(:))
        enableOut = 0;
    else
        enableOut = 1;
    end
    
    enable = enableOut;

== matlab function decoder/discreteDecode/HMM State Decoder/HMMStateDecoder ==
  data: stateLikelihoodsOut output; neural input size=[1 DecoderConstants.NUM_CONTINUOUS_CHANNELS]; clickStateOut output; decoderParams input Bus: decoderParams; stateLikelihoodsIn input; enable input; moveStateOut output; resetStateLikelihoods input double size=1; Z output; neuralMeans input size=[1 DecoderConstants.NUM_CONTINUOUS_CHANNELS]; xkin input; PxOut output
function [stateLikelihoodsOut, clickStateOut,moveStateOut, Z, PxOut] = HMMStateDecoder(neural, decoderParams, stateLikelihoodsIn, enable, resetStateLikelihoods, neuralMeans, xkin)
%% function that does the HMM work of the discrete decoder - 
%  calculates the state likelihoods based on state, neural data & transition probs
%%% SNF: multiclick ignores clickStateLikelihood, it's a single value and
%%% an artifact of non-dynamic programming from when there was only one
%%% click option. clickStateLikelihood is equal to one of the
%%% stateLikelihood entries. Likewise, moveStateLikelihood is always
%%% stateLikelihoods(1). For multiclick, we just use stateLikelihoods.  
%% define persistents and initialize 
persistent stateLikelihoods;
persistent clickStateLikelihood;
persistent moveStateLikelihood;
persistent latchedStateLikelihoodsIn;
persistent Zlatch;

if(isempty(clickStateLikelihood))
    stateLikelihoods            = stateLikelihoodsIn;
    latchedStateLikelihoodsIn   = stateLikelihoodsIn;
    %SNF points out that these commented lines below are the resetHMM states.
%     stateLikelihoods = zeros([double(DecoderConstants.MAX_DISCRETE_STATES) 1],'double');
%     stateLikelihoods(1) = 1;
    clickStateLikelihood        = 0;
    moveStateLikelihood         = 0;
    Zlatch                      = zeros(size(decoderParams.discreteProjector' * neural(:)),'double');
end
%% pull variables from the input decoderParams bus 
STATEVEC_SIZE = double(xkConstants.NUM_STATE_DIMENSIONS); 
numStates               = decoderParams.hmmNumStates; % SNF will check to see where this is assigned, it's initialized to 1
trans                   = decoderParams.hmmTrans;         % for buildHMM_multiclick this is calculated from the behavioral/training data. Others are hardcoded
emisMean                = decoderParams.hmmEmisMean;   % this is fit by buildHMM
emisCovarDet            = decoderParams.hmmEmisCovarDet;
emisCovarInv            = decoderParams.hmmEmisCovarInv;
stateModel              = decoderParams.hmmStateModel; % move-idle-click or move-idle or the multiclick variants of those 
projector               = decoderParams.discreteProjector;
invSoftNormVals         = decoderParams.discreteInvSoftNormVals;
pcaMeans                = decoderParams.discretePcaMeans;
hmmSpeedScalingEnable   = decoderParams.hmmSpeedScalingEnable;
hmmSpeedScalingBins     = decoderParams.hmmSpeedScalingBins;
hmmSpeedScalingPs       = decoderParams.hmmSpeedScalingPs;
dtMS                    = decoderParams.dtMS;
% CP - 2016-10-04 - means tracking is removed for discrete pathway
%meansTrackingEnable = decoderParams.discreteMeansTrackingEnable;
meansTrackingEnable     = false;
%% initialize transient variables- projector, distance and Px
projN = zeros(size(projector' * neural(:)),'double');
neuralDistance = zeros([double(DecoderConstants.MAX_DISCRETE_DECODE_CHANNELS) 1],'double');
Px = zeros([double(DecoderConstants.MAX_DISCRETE_STATES) 1],'double');
%% if the input has changed (i.e. a likelihood reset from the task), latch these values and update on the next enable
if resetStateLikelihoods %SNF says based on teh definitions in resetHMM shouldn't these be the resetLikelihoods? 
    latchedStateLikelihoodsIn = stateLikelihoodsIn;
end
%% new loop, enabled, run the thing: 
if enable
    % extract the previous values from the latched ones for no real reason (that SNF can see): 
    prevStateLikelihoods = latchedStateLikelihoodsIn;
    % do neural stuff if the settings say to: 
    neural(:) = neural(:) .* invSoftNormVals(:);
    if meansTrackingEnable
        neuralMeans(:) = neuralMeans(:) .* invSoftNormVals;
        neural(:) = neural(:) - neuralMeans(:) * double(dtMS);
    else
        neural(:) = neural(:) - pcaMeans(:);
    end
    projN = double(projector') * double(neural(:));
    Zlatch = projN;
    % do speed stuff if the settings say to: 
    if hmmSpeedScalingEnable
        % figure out what bin the current speed goes in
        currentSpeed = sqrt(sum(xkin(2:2:STATEVEC_SIZE).^2)); % now looks at all speeds. unused dimensions just have zeros
        speedInd = 1;
        for nsp = double(DecoderConstants.NUM_HMM_SPEED_BINS):-1:1
            if currentSpeed>hmmSpeedScalingBins(nsp)
                speedInd = nsp;
                break;
            end
        end
    end
%% Now calculate the likelihood for each state
    for s = 1:numStates
        emisMeanCur = squeeze(emisMean(s,:));
        emisCovarDetCur = emisCovarDet(s);
        emisCovarInvCur = squeeze(emisCovarInv(s,:,:));
        neuralDistance = projN(:)-emisMeanCur(:);
        %calculate the probablility of being in each state based on what
        %the neural data says
        Px(s) = (1/(emisCovarDetCur)^(0.5)) * ...
                exp(-0.5*(neuralDistance)' * emisCovarInvCur * (neuralDistance));
        if hmmSpeedScalingEnable
            Px(s) = Px(s) * hmmSpeedScalingPs(s,speedInd);
        end
    end
%% use those values to update the likelihoods: 
% multiply the transition matrix probabilities by prev state likelihoods and 
% the probability of going into the next state based on what the neural data says
    stateLikelihoods = trans * prevStateLikelihoods .* Px(:);
    stateLikelihoods = stateLikelihoods / sum(stateLikelihoods); 
%% backup plan for before decoder is completely initialized - just set the first state to 1
    if any(isnan(stateLikelihoods))
        stateLikelihoods=zeros(size(stateLikelihoods));
        stateLikelihoods(1)=1;
    end
%% assign the likelihoods we just established to the latched case for the next round 
    latchedStateLikelihoodsIn = stateLikelihoods;
end
%% assign the proper outputs based on the stateModel
% click and move state are defined as size 1. Using stateLikelihoods
% instead for multiclick (hint: these get used in getClickState among other places) 
% this is always true. *and always will be* (hear me, future coders?) -SNF:
moveStateLikelihood = stateLikelihoods(1);
switch stateModel
    case DiscreteStates.STATE_MODEL_MOVECLICK
        clickStateLikelihood = stateLikelihoods(2);
    case DiscreteStates.STATE_MODEL_MOVEIDLECLICK
        clickStateLikelihood = stateLikelihoods(3);
%%% cases for multiclick model- entry in likelihoods matrix for
%%% click determined by click target. move is still 1. yay. 
%     case DiscreteStates.STATE_MODEL_MULTICLICK
%         moveStateLikelihood = stateLikelihoods(1);
%     case DiscreteStates.STATE_MODEL_MULTICLICK3
%         moveStateLikelihood = stateLikelihoods(1);
end
%% assign the outputs
PxOut               = Px(:);
clickStateOut       = clickStateLikelihood;
moveStateOut        = moveStateLikelihood;
stateLikelihoodsOut = stateLikelihoods;
Z                   = Zlatch;
